simulink model "robust_control"  (R2025b)
settings: Solver=VariableStepAuto  StartTime=0.0  StopTime=Tf  FixedStep=0.01  RelTol=1e-3  EnableMultiTasking=on
values from neighbouring files (symbols this model uses):
  D = [zeros(n, n); eye(n)]    [main.m]
  Kd = 5 * eye(n)    [main.m]
  Kp = 25 * eye(n)    [main.m]
  Q = lyap(H_tilde, P)    [main.m]
  qi = [0; pi/4]    [main.m]
  ro = 70    [main.m]
  Tc = 0.005    [main.m]
settings Model: Creator=donato  LastModifiedBy=simy
settings SolverCC: AlgebraicLoopSolver=TrustRegion
settings DataIOCC: ReturnWorkspaceOutputs=off
settings OptimizationCC: LifeSpan=inf
settings DebuggingCC: UnconnectedInputMsg=warning  UnconnectedOutputMsg=warning  UnconnectedLineMsg=warning  SFUnexpectedBacktrackingDiag=warning  SFNoUnconditionalDefaultTransitionDiag=warning  SFExecutionAtInitializationDiag=none  ArithmeticOperatorsInVariantConditions=warning
settings ModelReferenceCC: EnableRefExpFcnMdlSchedulingChecks=on
settings SFSimCC: SimUseLocalCustomCode=off  CustomCodeUndefinedFunction=UseInterfaceOnly
settings RTWCC: RTWUseLocalCustomCode=off  GPUComputeCapability=3.5
settings CodeAppCC: StateflowObjectComments=on
settings GRTTargetCC: TargetLangStandard=C89/C90 (ANSI)
settings ConfigComp: CovMetricSettings=dw  CovSaveCumulativeToWorkspaceVar=on  CovSaveSingleToWorkspaceVar=on  CovExternalEMLEnable=off

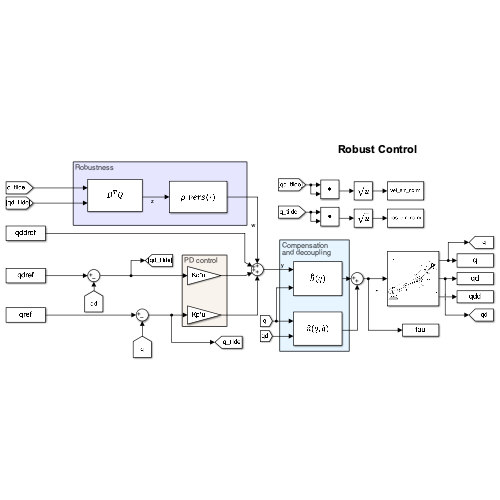
[thumbnail: Simulink's stored preview of the top-level diagram]
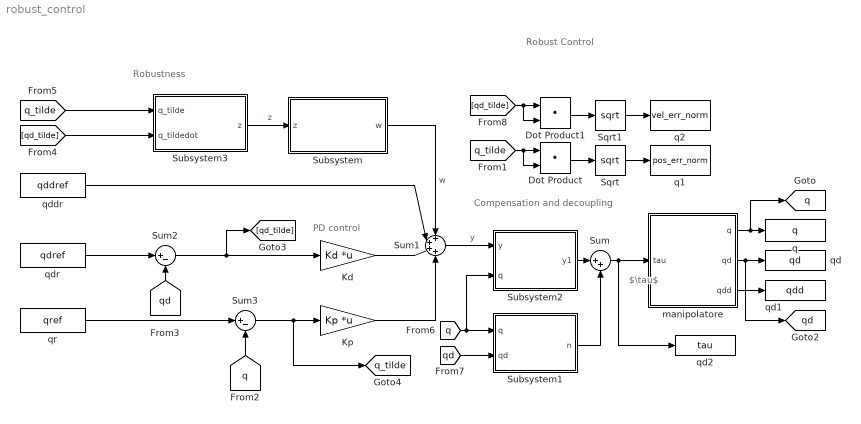
== system robust_control ==
  note: Compensation
      | and decoupling
  note: PD control
  note: Robustness
  note: $\tau$
  note: Robust Control
  Dot Product : DotProduct  OutDataTypeStr=Inherit: Inherit via internal rule
  Dot Product1 : DotProduct  OutDataTypeStr=Inherit: Inherit via internal rule
  Kd : Gain  Gain=Kd  Multiplication=Matrix(K*u)
  Kp : Gain  Gain=Kp  Multiplication=Matrix(K*u)
  Sqrt : Sqrt
  Sqrt1 : Sqrt
  Subsystem : Subsystem
      mask Display: image('ro.png');
  Subsystem1 : Subsystem
      mask Display: image('n.png');
  Subsystem2 : Subsystem
      mask Display: image('B.png');
  Subsystem3 : Subsystem
      mask Display: image('dq.png');
  Sum : Sum  Inputs=|++
  Sum1 : Sum  Inputs=++++
  Sum2 : Sum  Inputs=|+-
  Sum3 : Sum  Inputs=|+-
  manipolatore : Subsystem
      mask Display: image('manipolatore.png', [0,0,0,0,95,100]);
  q : ToWorkspace  VariableName=q  SampleTime=Tc
  q1 : ToWorkspace  VariableName=pos_err_norm  SampleTime=Tc
  q2 : ToWorkspace  VariableName=vel_err_norm  SampleTime=Tc
  qd : ToWorkspace  VariableName=qd  SampleTime=Tc
  qd1 : ToWorkspace  VariableName=qdd  SampleTime=Tc
  qd2 : ToWorkspace  VariableName=tau  SampleTime=Tc
  qddr : FromWorkspace  VariableName=qddref  SampleTime=Tc
  qdr : FromWorkspace  VariableName=qdref  SampleTime=Tc
  qr : FromWorkspace  VariableName=qref  SampleTime=Tc
  tag scope: q=global, q_tilde=global, qd=global
  wires:
  Sum1/1 -> Subsystem2/1(y)  "y"
  Sum3/1 -> [q_tilde], Kp/1
  Sum2/1 -> [qd_tilde], Kd/1
  qr/1 -> Sum3/1
  qdr/1 -> Sum2/1
  Kp/1 -> Sum1/4
  Kd/1 -> Sum1/3
  qddr/1 -> Sum1/2
  [q] -> Sum3/2
  [qd] -> Sum2/2
  Sum/1 -> qd2/1, manipolatore/1(tau)
  Subsystem/1(w) -> Sum1/1  "w"
  [q] -> Subsystem1/1(q), Subsystem2/2(q)
  [qd] -> Subsystem1/2(qd)
  Subsystem1/1(n) -> Sum/2
  Subsystem2/1(y1) -> Sum/1
  [q_tilde] -> Subsystem3/1(q_tilde)
  [qd_tilde] -> Subsystem3/2(q_tildedot)
  Subsystem3/1(z) -> Subsystem/1(z)  "z"
  manipolatore/1(q) -> q/1, [q]
  manipolatore/2(qd) -> qd/1, [qd]
  manipolatore/3(qdd) -> qd1/1
  Dot Product/1 -> Sqrt/1
  Sqrt/1 -> q1/1
  [q_tilde] -> Dot Product/2, Dot Product/1
  Sqrt1/1 -> q2/1
  Dot Product1/1 -> Sqrt1/1
  [qd_tilde] -> Dot Product1/2, Dot Product1/1

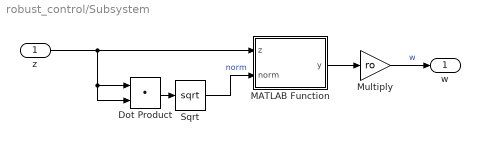
== system robust_control/Subsystem ==
  z : Inport
  Dot Product : DotProduct  OutDataTypeStr=Inherit: Inherit via internal rule
  MATLAB Function : MATLAB Function  TreatAsAtomicUnit=on
  Multiply : Gain  Gain=ro
  Sqrt : Sqrt
  w : Outport
  wires:
  Sqrt/1 -> MATLAB Function/2(norm)  "norm"
  Multiply/1 -> w/1  "w"
  Dot Product/1 -> Sqrt/1
  z/1 -> Dot Product/2, Dot Product/1, MATLAB Function/1(z)
  MATLAB Function/1(y) -> Multiply/1

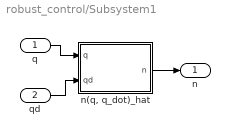
== system robust_control/Subsystem1 ==
  q : Inport
  qd : Inport  Port=2
  "n(q, q_dot)_hat" : MATLAB Function  TreatAsAtomicUnit=on
  n : Outport
  wires:
  q/1 -> "n(q, q_dot)_hat"/1(q)
  "n(q, q_dot)_hat"/1(n) -> n/1
  qd/1 -> "n(q, q_dot)_hat"/2(qd)

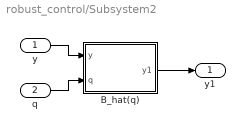
== system robust_control/Subsystem2 ==
  y : Inport
  q : Inport  Port=2
  B_hat(q) : MATLAB Function  TreatAsAtomicUnit=on
  y1 : Outport
  wires:
  q/1 -> B_hat(q)/2(q)
  B_hat(q)/1(y1) -> y1/1
  y/1 -> B_hat(q)/1(y)

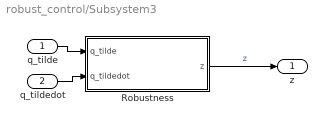
== system robust_control/Subsystem3 ==
  q_tilde : Inport
  q_tildedot : Inport  Port=2
  Robustness : MATLAB Function  TreatAsAtomicUnit=on
  z : Outport
  wires:
  q_tildedot/1 -> Robustness/2(q_tildedot)
  Robustness/1(z) -> z/1  "z"
  q_tilde/1 -> Robustness/1(q_tilde)

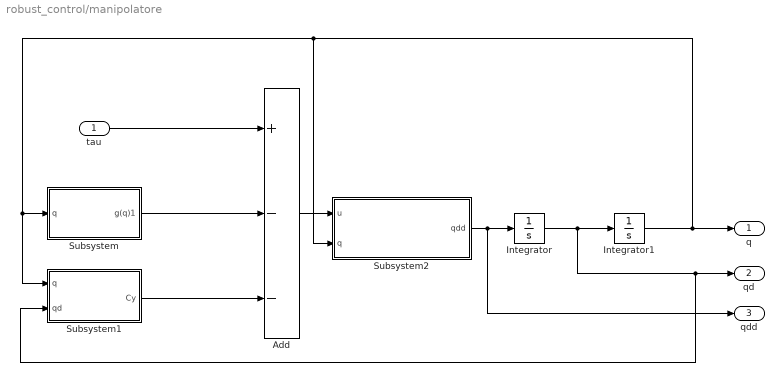
== system robust_control/manipolatore ==
  tau : Inport
  Add : Sum  Inputs=+--
  Integrator : Integrator  InitialCondition=[0;0]
  Integrator1 : Integrator  InitialCondition=qi
  Subsystem : Subsystem
      mask Display: image('g.png');
  Subsystem1 : Subsystem
      mask Display: image('C.png');
  Subsystem2 : Subsystem
      mask Display: image('inv_dinamica.png', [0,0,0,0,90,90]);
  q : Outport
  qd : Outport  Port=2
  qdd : Outport  Port=3
  wires:
  Integrator/1 -> Integrator1/1, Subsystem1/2(qd), qd/1
  Integrator1/1 -> q/1, Subsystem2/2(q), Subsystem/1(q), Subsystem1/1(q)
  tau/1 -> Add/1
  Subsystem/1(g(q)1) -> Add/2
  Subsystem1/1(Cy) -> Add/3
  Subsystem2/1(qdd) -> Integrator/1, qdd/1
  Add/1 -> Subsystem2/1(u)

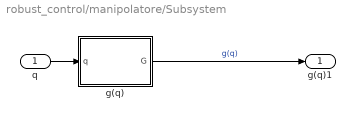
== system robust_control/manipolatore/Subsystem ==
  q : Inport
  g(q) : MATLAB Function  TreatAsAtomicUnit=on
  g(q)1 : Outport
  wires:
  g(q)/1(G) -> g(q)1/1  "g(q)"
  q/1 -> g(q)/1(q)

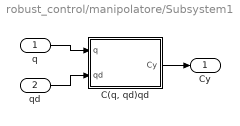
== system robust_control/manipolatore/Subsystem1 ==
  q : Inport
  qd : Inport  Port=2
  "C(q, qd)qd" : MATLAB Function  TreatAsAtomicUnit=on
  Cy : Outport
  wires:
  "C(q, qd)qd"/1(Cy) -> Cy/1
  qd/1 -> "C(q, qd)qd"/2(qd)
  q/1 -> "C(q, qd)qd"/1(q)

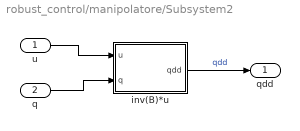
== system robust_control/manipolatore/Subsystem2 ==
  u : Inport
  q : Inport  Port=2
  inv(B)*u : MATLAB Function  TreatAsAtomicUnit=on
  qdd : Outport
  wires:
  inv(B)*u/1(qdd) -> qdd/1  "qdd"
  q/1 -> inv(B)*u/2(q)
  u/1 -> inv(B)*u/1(u)

== matlab function robust_control/Subsystem/MATLAB Function ==
  data: z input; norm input; y output; eps parameter
function y = fcn(z, norm, eps)
    if norm >= eps
        y = z / norm;
    else
        y = z / eps;
    end
end

== matlab function robust_control/Subsystem3/Robustness ==
  data: q_tilde input; z output; q_tildedot input; D parameter; Q parameter
function z = fcn(q_tilde, q_tildedot, D, Q)
    eps = [q_tilde; q_tildedot];
    z = D' * Q * eps;
end

== matlab function robust_control/Subsystem2/B_hat(q) ==
  data: y input; y1 output; q input
function y1 = fcn(y, q)
    a1 = 1; l1 = 0.5; l2 = 0.5; ml1 = 50; ml2 = 50; Il1 = 10; Il2 = 10; 
    kr1 = 100; kr2 = 100; mm2 = 5; Im1 = 0.01; Im2 = 0.01; 

    % INERTIA MATRIX
    b11 = Il1 + ml1 * l1^2 + kr1^2 * Im1 + Il2 + ml2 * (a1^2 + l2^2) ...
         + Im2 + mm2 * a1^2;
    b12 = Il2 + ml2 * l2^2 + kr2 * Im2;
    b21 = b12;
    b22 = Il2 + ml2 * l2^2 + kr2^2 * Im2;
    B = [b11 b12; 
         b21 b22];

    y1 = B * y;
end

== matlab function robust_control/Subsystem1/n(q, q_dot)_hat ==
  data: q input; n output; qd input
function n = fcn(q, qd)
    a1 = 1; l1 = 0.5; l2 = 0.5; ml1 = 50; ml2 = 50; mm2 = 5; g = 9.81; 
    teta1 = q(1); teta2 = q(2); c1 = cos(teta1); c12 = cos(teta1 + teta2);

    g1 = (ml1 * l1 + mm2 * a1 + ml2 * a1) * g * c1 + ml2 * l2 * g * c12;
    g2 = ml2 * l2 * g * c12;
    G = [g1; 
         g2];

    n = G;
end

== matlab function robust_control/manipolatore/Subsystem/g(q) ==
  data: q input; G output size=[2, 1]
function G = fcn(q)
    
    a1 = 1; l1 = 0.5; l2 = 0.5; ml1 = 50; ml2 = 50; mm2 = 5; g = 9.81; 
    teta1 = q(1); teta2 = q(2); c1 = cos(teta1); c12 = cos(teta1 + teta2);

    g1 = (ml1 * l1 + mm2 * a1 + ml2 * a1) * g * c1 + ml2 * l2 * g * c12;
    g2 = ml2 * l2 * g * c12;
    G = [g1;
         g2];
end

== matlab function robust_control/manipolatore/Subsystem1/C(q, qd)qd ==
  data: q input; Cy output size=[2, 1]; qd input
function Cy = fcn(q, qd)
    a1 = 1; l2 = 0.5; ml2 = 50; 
    teta2 = q(2); teta1d = qd(1); teta2d = qd(2); s2 = sin(teta2); 

    h = -ml2 * a1 * l2 * s2;
    C = [h*teta2d h*(teta1d+teta2d); -h*teta1d 0];
    Cy = C * qd;
end

== matlab function robust_control/manipolatore/Subsystem2/inv(B)*u ==
  data: u input; qdd output size=[2, 1]; q input
function qdd = fcn(u, q)
    a1 = 1; l1 = 0.5; l2 = 0.5; ml1 = 50; ml2 = 50; Il1 = 10; Il2 = 10; 
    kr1 = 100; kr2 = 100; mm2 = 5; Im1 = 0.01; Im2 = 0.01;

    teta2 = q(2); c2 = cos(teta2); 

    b11 = Il1 + ml1 * l1^2 + kr1^2 * Im1 + Il2 + ...
          ml2 * (a1^2 + l2^2 + 2 * a1 * l2 *c2) + Im2 + mm2 * a1^2;
    b12 = Il2 + ml2 * (l2^2 + a1 * l2 * c2) + kr2 * Im2;
    b21 = b12;
    b22 = Il2 + ml2 * l2^2 + kr2^2 * Im2;
    B = [b11 b12; b21 b22];

    qdd = B\u;
end
